simulink model "selector_port_test_tmp"  (Simulink 8.3)
settings: Solver=VariableStepDiscrete  StartTime=0.0  StopTime=0  MaxStep=1  RelTol=1e-3
settings Model: Creator=arnaud  LastModifiedBy=hbourbou
settings DataIOCC: ExternalInput=xin  SaveFormat=Structure
settings OptimizationCC: ExpressionDepthLimit=2147483647
settings DebuggingCC: FcnCallInpInsideContextMsg=EnableAllAsWarning  FrameProcessingCompatibilityMsg=error

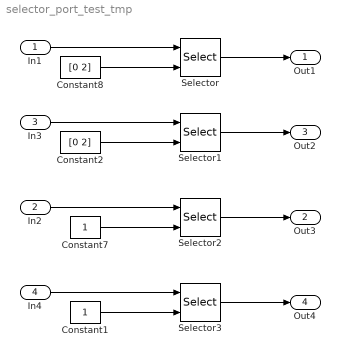
== system selector_port_test_tmp ==
  In1 : Inport  PortDimensions=3
  In2 : Inport  Port=2  PortDimensions=3
  In3 : Inport  Port=3  PortDimensions=3
  In4 : Inport  Port=4  PortDimensions=3
  Constant1 : Constant
  Constant2 : Constant  Value=[0 2]
  Constant7 : Constant
  Constant8 : Constant  Value=[0 2]
  Selector : Selector  IndexMode=Zero-based  InputPortWidth=3  IndexOptions=Index vector (port)  Indices=[1 0 0]  OutputSizes=1
  Selector1 : Selector  IndexMode=Zero-based  InputPortWidth=3  IndexOptions=Index vector (port)  Indices=[1 0 0]  OutputSizes=1
  Selector2 : Selector  InputPortWidth=3  IndexOptions=Index vector (port)  Indices=2  OutputSizes=1
  Selector3 : Selector  IndexMode=Zero-based  InputPortWidth=3  IndexOptions=Index vector (port)  Indices=2  OutputSizes=2
  Out1 : Outport
  Out3 : Outport  Port=2
  Out2 : Outport  Port=3
  Out4 : Outport  Port=4
  wires:
  Selector/1 -> Out1/1
  In1/1 -> Selector/1
  Selector2/1 -> Out3/1
  In2/1 -> Selector2/1
  Constant8/1 -> Selector/2
  Constant7/1 -> Selector2/2
  Selector1/1 -> Out2/1
  In3/1 -> Selector1/1
  Selector3/1 -> Out4/1
  In4/1 -> Selector3/1
  Constant2/1 -> Selector1/2
  Constant1/1 -> Selector3/2
